simulink model "led"  (R2022a)
settings: Solver=FixedStepAuto  StartTime=0.0  StopTime=10.0  RelTol=1e-3  EnableMultiTasking=on
libraries: mbedblockslib x1
settings Model: ExtModeTrigDuration=10  Creator=MATLAB  LastModifiedBy=FUGAZI
settings OptimizationCC: EnhancedBackFolding=on  PassReuseOutputArgsAs=Individual arguments  ZeroExternalMemoryAtStartup=off  ZeroInternalMemoryAtStartup=off  MaxStackSize=64  OptimizeBlockOrder=speed  DifferentSizesBufferReuse=on  OptimizationCustomize=off  EfficientTunableParamExpr=on
settings DebuggingCC: ParameterTunabilityLossMsg=error
settings HardwareCC: ProdBitPerPointer=32  ProdBitPerSizeT=32  ProdBitPerPtrDiffT=32  ProdLargestAtomicInteger=Long  ProdLargestAtomicFloat=Double  ProdWordSize=32  ProdLongLongMode=on  ProdHWDeviceType=ARM Compatible->ARM Cortex
settings SFSimCC: MATLABDynamicMemAlloc=off
settings RTWCC: SystemTargetFile=ert.tlc  HardwareBoard=STM32 Nucleo L476RG  TemplateMakefile=ert_default_tmf  Toolchain=GNU Tools for ARM Embedded Processors
settings CodeAppCC: ForceParamTrailComments=on  IgnoreCustomStorageClasses=off  OperatorAnnotations=on  SimulinkDataObjDesc=on  SFDataObjDesc=on  InsertBlockDesc=on
settings ERTTargetCC: ExtModeTransport=3  ExtModeStaticAlloc=on  ExtModeStaticAllocSize=2000  ExtModeMexFile=ext_xcp  ExtModeIntrfLevel=Level2 - Open

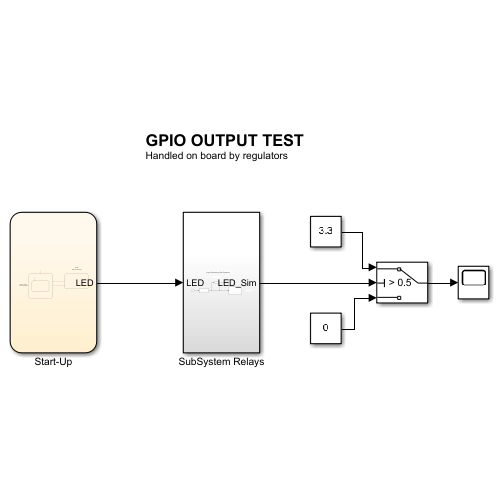
[thumbnail: Simulink's stored preview of the top-level diagram]
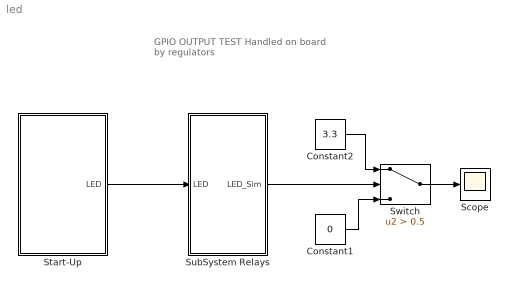
== system led ==
  note: GPIO OUTPUT TEST
      | Handled on board by regulators
  Constant1 : Constant  Value=0
  Constant2 : Constant  Value=3.3
  Scope : Scope
  Start-Up : Stateflow chart  TreatAsAtomicUnit=on
  SubSystem Relays : Subsystem
  Switch : Switch  Criteria=u2 > Threshold  Threshold=0.5  SaturateOnIntegerOverflow=off  InputSameDT=off
  wires:
  Constant2/1 -> Switch/1
  SubSystem Relays/1(LED_Sim) -> Switch/2
  Constant1/1 -> Switch/3
  Switch/1 -> Scope/1
  Start-Up/1(LED) -> SubSystem Relays/1(LED)

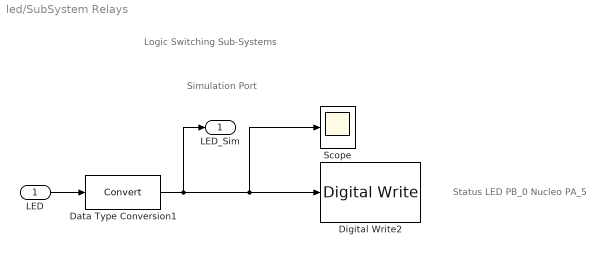
== system led/SubSystem Relays ==
  note: Logic Switching Sub-Systems
  note: Simulation Port
  note: Status LED PB_0
      | Nucleo PA_5
  LED : Inport
  Data Type Conversion1 : DataTypeConversion  SaturateOnIntegerOverflow=off  RndMeth=Floor
  Digital Write2 : mbedblockslib/Digital Write  Pin=PA_5  Direction=output
      settings: SourceProductBaseCode=MICROBIT,NUCLEO,STMICRODIS
  Scope : Scope
  LED_Sim : Outport
  wires:
  LED/1 -> Data Type Conversion1/1
  Data Type Conversion1/1 -> Digital Write2/1, Scope/1, LED_Sim/1

== stateflow chart led/Start-Up ==
  note: TEST:
      | Routine Checks
  state Run % Parent
    state LED % Child
      entry: % none
      LED = 1; % LED On
      exit: % none
    (default) -> LED % Child
  state Check % Check Sub-Systems
    entry:
    LED = 0; % LED Off
    exit:
  note: Check Input
      | Power present?
  (default) -> Run % Parent
  Check % Check Sub-Systems -> Run % Parent : after(2,sec)
  Run % Parent -> Check % Check Sub-Systems : after(2,sec)
  data: LED output
